simulink model "chap7_1sim"  (Simulink 7.0)
settings: Solver=ode45  StartTime=0.0  StopTime=10  FixedStep=0.001  RelTol=1e-3
settings Model: Creator=Administrator  LastModifiedBy=eleliuj  ExtModeTrigMode=oneshot  ExtModeArmWhenConnect=off
settings DataIOCC: LimitDataPoints=off  SignalLoggingName=sigsOut
settings OptimizationCC: BooleanDataType=off
settings DebuggingCC: SaveWithParameterizedLinksMsg=none  SignalResolutionControl=TryResolveAllWithWarning  SolverPrmCheckMsg=none  MultiTaskDSMMsg=warning  MultiTaskCondExecSysMsg=none  StrictBusMsg=None
settings HardwareCC: TargetUnknown=on
settings RTWCC: IncludeERTFirstTime=on
settings GRTTargetCC: TargetFcnLib=ansi_tfl_tmw.mat

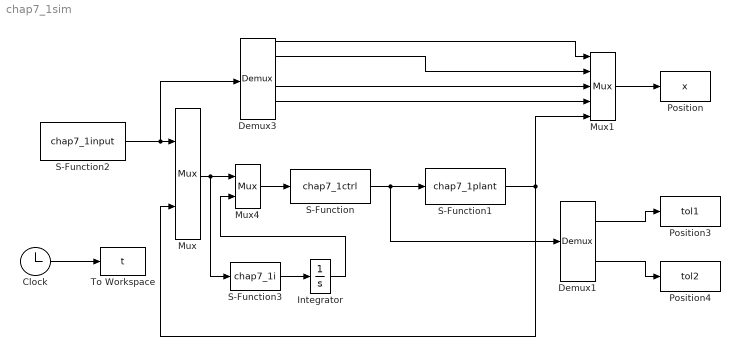
== system chap7_1sim ==
  Clock : Clock
      settings: Decimation=10
  Demux1 : Demux  Outputs=2
  Demux3 : Demux  Outputs=6
  Integrator : Integrator
  Mux : Mux  Inputs=2
  Mux1 : Mux  Inputs=5
  Mux4 : Mux  Inputs=2
  Position : ToWorkspace  VariableName=x  SampleTime=-1  SaveFormat=Array
  Position3 : ToWorkspace  VariableName=tol1  SampleTime=-1  SaveFormat=Array
  Position4 : ToWorkspace  VariableName=tol2  SampleTime=-1  SaveFormat=Array
  S-Function : S-Function  FunctionName=chap7_1ctrl
  S-Function1 : S-Function  FunctionName=chap7_1plant
  S-Function2 : S-Function  FunctionName=chap7_1input
  S-Function3 : S-Function  FunctionName=chap7_1i
  To Workspace : ToWorkspace  VariableName=t  SampleTime=-1  SaveFormat=Array
  wires:
  Mux/1 -> S-Function3/1, Mux4/1
  S-Function1/1 -> Mux/2, Mux1/5
  S-Function2/1 -> Demux3/1, Mux/1
  Demux1/1 -> Position3/1
  Demux1/2 -> Position4/1
  Mux1/1 -> Position/1
  S-Function/1 -> S-Function1/1, Demux1/1
  Mux4/1 -> S-Function/1
  S-Function3/1 -> Integrator/1
  Integrator/1 -> Mux4/2
  Clock/1 -> To Workspace/1
  Demux3/4 -> Mux1/3
  Demux3/5 -> Mux1/4
  Demux3/1 -> Mux1/1
  Demux3/2 -> Mux1/2
